simulink model "pdref"  (Simulink 6.2)
settings: Solver=ode23s  StartTime=0.0  StopTime=100  RelTol=1e-3
values from neighbouring files (symbols this model uses):
  g = 9.81    [bipedparams.m]
  st = 0.005    [bipedparams.m]    (also in pdparams.m)
libraries: bipedlib x2, simulink x1
settings Model: LastModifiedBy=Olli Haavisto  BufferReuse=off
settings DataIOCC: SaveFormat=StructureWithTime  SaveOutput=off  SaveTime=off  SignalLoggingName=sigsOut
settings OptimizationCC: InlineInvariantSignals=on  OptimizeBlockIOStorage=off  BufferReuse=off  ExpressionFolding=off  LocalBlockOutputs=off
settings DebuggingCC: CheckMatrixSingularityMsg=warning  UnnecessaryDatatypeConvMsg=warning  SignalLabelMismatchMsg=warning  SFcnCompatibilityMsg=warning
settings HardwareCC: TargetUnknown=on

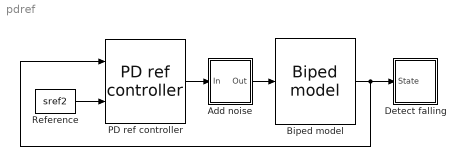
== system pdref ==
  Add noise : Subsystem
  Biped model : bipedlib/Biped model  robot=robot  initstate=initstate  knees=knees  groundp=groundp  g=g  st=st
  Detect falling : Subsystem
  PD ref controller : bipedlib/PD ref controller
  Reference : FromWorkspace  VariableName=sref2  SampleTime=st  Interpolate=off  OutputAfterFinalValue=Cyclic repetition
  wires:
  PD ref controller/1 -> Add noise/1(In)
  Reference/1 -> PD ref controller/2
  Add noise/1(Out) -> Biped model/1
  Biped model/1 -> Detect falling/1(State), PD ref controller/1

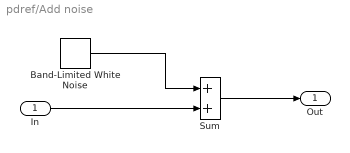
== system pdref/Add noise ==
  In : Inport  Port=1  LatchInput=off
  Band-Limited White Noise : simulink/Sources/Band-Limited White Noise  Cov=[1 1 1 1]*0.01  Ts=st  seed=[23 3 4 1]
  Sum : Sum  SaturateOnIntegerOverflow=on
  Out : Outport
  wires:
  Sum/1 -> Out/1
  In/1 -> Sum/2
  Band-Limited White Noise/1 -> Sum/1

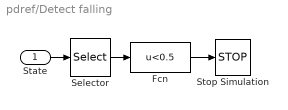
== system pdref/Detect falling ==
  State : Inport  Port=1  LatchInput=off
  Fcn : Fcn  Expr=u<0.5
  Selector : Selector  Elements=[2]  InputPortWidth=16
  Stop Simulation : Stop
  wires:
  State/1 -> Selector/1
  Selector/1 -> Fcn/1
  Fcn/1 -> Stop Simulation/1
